simulink model "random_signal"  (R2022b)
settings: Solver=VariableStepAuto  StartTime=0.0  StopTime=100  RelTol=1e-3
values from neighbouring files (symbols this model uses):
  Wd = c2d(W, T0)    [my_hist.m]
settings Model: Creator=mrxmi  LastModifiedBy=mrxmi

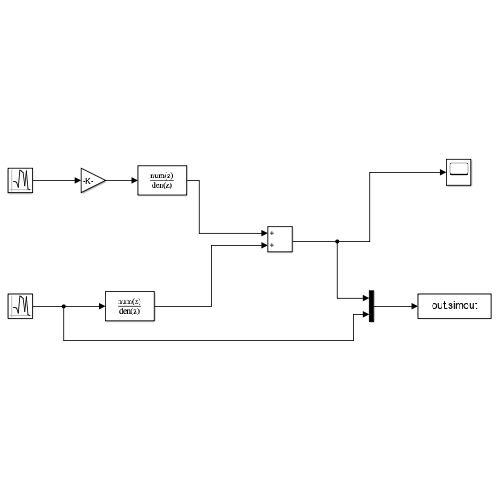
[thumbnail: Simulink's stored preview of the top-level diagram]
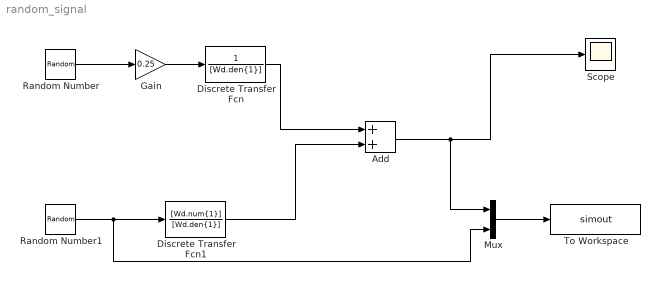
== system random_signal ==
  Add : Sum
  Discrete Transfer Fcn : DiscreteTransferFcn  Denominator=[Wd.den{1}]
  Discrete Transfer Fcn1 : DiscreteTransferFcn  Numerator=[Wd.num{1}]  Denominator=[Wd.den{1}]
  Gain : Gain  Gain=0.25
  Mux : Mux  Inputs=2
  Random Number : RandomNumber  Seed=1  SampleTime=0.1
  Random Number1 : RandomNumber  SampleTime=0.1
  Scope : Scope
  To Workspace : ToWorkspace  VariableName=simout  SaveFormat=Structure With Time  SampleTime=-1
  wires:
  Random Number/1 -> Gain/1
  Gain/1 -> Discrete Transfer Fcn/1
  Random Number1/1 -> Mux/2, Discrete Transfer Fcn1/1
  Discrete Transfer Fcn1/1 -> Add/2
  Discrete Transfer Fcn/1 -> Add/1
  Add/1 -> Mux/1, Scope/1
  Mux/1 -> To Workspace/1
